simulink model "hibrido"  (R2020a)
settings: Solver=VariableStepAuto  StartTime=0.0  StopTime=3  RelTol=1e-3
values from neighbouring files (symbols this model uses):
  fd = [10/sqrt(2); 10/sqrt(2)]    [hibrido_control.m]
  Ke = 1000    [hibrido_control.m]
  Kp = wn_c^2*eye(2)    [hibrido_control.m]
  Kpf = wn_f^2    (= 16000000)    [hibrido_control.m]
  Kv = 2*xi*wn_c*eye(2)    [hibrido_control.m]
  Kvf = 2*xi*wn_f    (= 8000)    [hibrido_control.m]
  tstep = 0.2    [hibrido_control.m]
  x0 = [0.5, 1.5]    [hibrido_control.m]
  xf = [1.5, 0.5]    [hibrido_control.m]
undefined symbols (not defined in the file or in its folder): coriolis, Robot
libraries: roblocks x14
settings Model: Creator=User  LastModifiedBy=USUARIO
settings SFSimCC: CustomCodeUndefinedFunction=UseInterfaceOnly

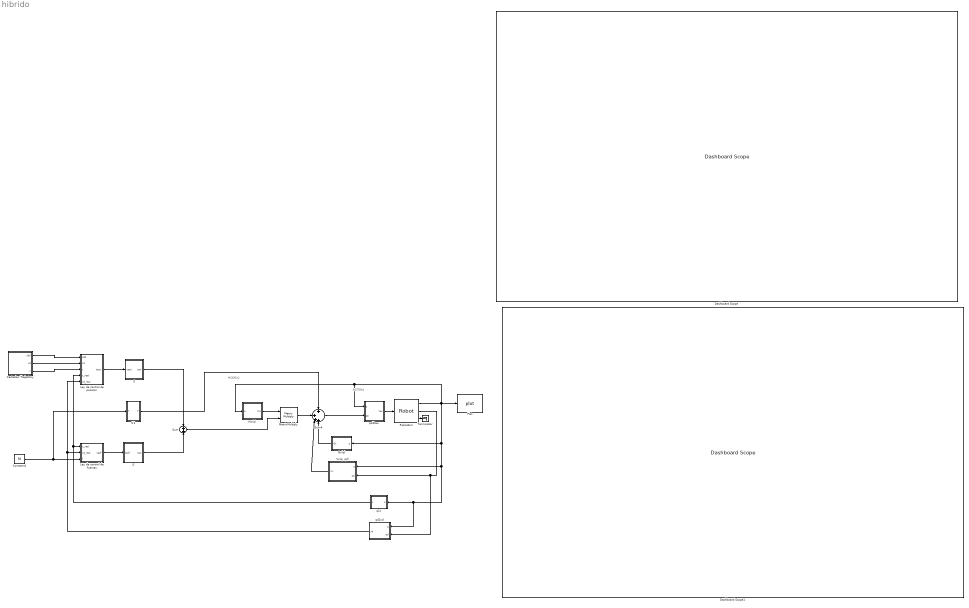
== system hibrido ==
  note: SISTEMA
  note: MODELO
  Cartesian Trajectory : Subsystem  mask{initial_x=x0, final_x=xf, t_max=tf, ts=tstep}
      mask prompts: initial_x "Initial X"; final_x "Final X"; t_max "Maximum time"; ts "Timestep"
  Constant1 : Constant  Value=fd
  Dashboard Scope : DashboardScope
  Dashboard Scope1 : DashboardScope  Ymax=13
  "Gx(q) " : Subsystem  mask{robot=Robot}
  Ley de control de fuerzas : Subsystem
  Ley de control de posicion : Subsystem
  MatrixMultiply : Product  Multiplication=Matrix(*)
  Mx(q) : Subsystem  mask{robot=Robot}
  Plot : roblocks/Arm/plot  robot=Robot  fps=30  holdplot=on
  RobotArm : roblocks/Arm/Robot  robot=Robot  q0=q0
  S : Subsystem  mask{robot=0}
  S' : Subsystem  mask{robot=0}
  S'1 : Subsystem  mask{robot=0}
  Sum : Sum  Inputs=+|+
  Sum4 : Sum  Inputs=+|+++
  Terminator : Terminator
  "Vx(q, qd)" : Subsystem  mask{robot=Robot}
  psi2tau : Subsystem  mask{robot=Robot}
  q2x : Subsystem  mask{robot=Robot}
  qd2xd : Subsystem  mask{robot=Robot}
  wires:
  RobotArm/3 -> Terminator/1
  Sum4/1 -> psi2tau/2(psi)
  RobotArm/1 -> qd2xd/1(q), q2x/1(q), "Vx(q, qd)"/1(q), "Gx(q) "/1(q), Plot/1, Mx(q)/1(q), psi2tau/1(q)
  RobotArm/2 -> qd2xd/2(qd), "Vx(q, qd)"/2(qd)
  Mx(q)/1(Mx) -> MatrixMultiply/1
  psi2tau/1(tau) -> RobotArm/1
  Cartesian Trajectory/1(xdd) -> Ley de control de posicion/1(xdd)
  Cartesian Trajectory/2(xd) -> Ley de control de posicion/2(xd)
  Cartesian Trajectory/3(x) -> Ley de control de posicion/3(x)
  q2x/1(x) -> Ley de control de posicion/4(x_real), Ley de control de fuerzas/1(x_real)
  qd2xd/1(xd) -> Ley de control de posicion/5(xd_real), Ley de control de fuerzas/2(xd_real)
  Constant1/1 -> S'1/1(f), Ley de control de fuerzas/3(f)
  Ley de control de posicion/1(taoc') -> S/1(taoc')
  Ley de control de fuerzas/1(taof') -> S'/1(taof')
  S/1(tao') -> Sum/1
  S'/1(tao') -> Sum/2
  Sum/1 -> MatrixMultiply/2
  MatrixMultiply/1 -> Sum4/2
  "Gx(q) "/1(Gx) -> Sum4/4
  "Vx(q, qd)"/1(Vx) -> Sum4/3
  S'1/1(f') -> Sum4/1

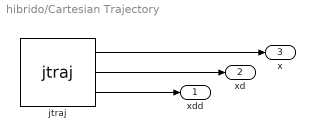
== system hibrido/Cartesian Trajectory ==
  jtraj : roblocks/Toolbox/jtraj  q0=initial_x  qf=final_x  tmax=t_max  ts=ts
  xdd : Outport  VectorParamsAs1DForOutWhenUnconnected=off
  xd : Outport  Port=2  VectorParamsAs1DForOutWhenUnconnected=off
  x : Outport  Port=3  VectorParamsAs1DForOutWhenUnconnected=off
  wires:
  jtraj/2 -> xd/1
  jtraj/1 -> x/1
  jtraj/3 -> xdd/1

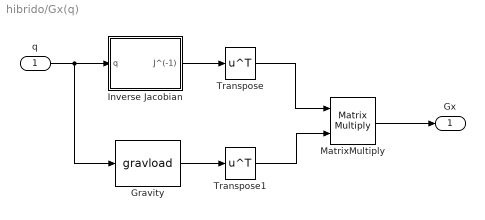
== system hibrido/Gx(q)  ==
  q : Inport
  Gravity : roblocks/Arm/gravload  robot=Robot
  Inverse Jacobian : Subsystem  mask{robot=robot}
  MatrixMultiply : Product  Multiplication=Matrix(*)
  Transpose : Math  Operator=transpose  SignedPower=on  SaturateOnIntegerOverflow=on
  Transpose1 : Math  Operator=transpose  SignedPower=on  SaturateOnIntegerOverflow=on
  Gx : Outport  VectorParamsAs1DForOutWhenUnconnected=off
  wires:
  q/1 -> Gravity/1, Inverse Jacobian/1(q)
  Inverse Jacobian/1(J^(-1)) -> Transpose/1
  Transpose/1 -> MatrixMultiply/1
  Gravity/1 -> Transpose1/1
  MatrixMultiply/1 -> Gx/1
  Transpose1/1 -> MatrixMultiply/2

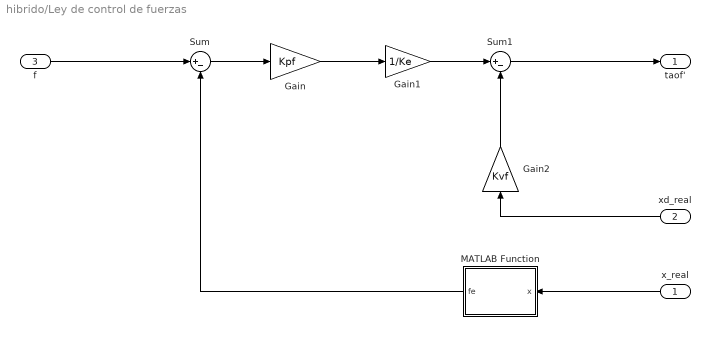
== system hibrido/Ley de control de fuerzas ==
  x_real : Inport
  xd_real : Inport  Port=2
  f : Inport  Port=3
  Gain : Gain  Gain=Kpf
  Gain1 : Gain  Gain=1/Ke
  Gain2 : Gain  Gain=Kvf
  MATLAB Function : MATLAB Function  TreatAsAtomicUnit=on
  Sum : Sum  Inputs=|+-
  Sum1 : Sum  Inputs=|+-
  taof' : Outport
  wires:
  Gain1/1 -> Sum1/1
  Gain2/1 -> Sum1/2
  Sum/1 -> Gain/1
  Sum1/1 -> taof'/1
  Gain/1 -> Gain1/1
  x_real/1 -> MATLAB Function/1(x)
  xd_real/1 -> Gain2/1
  f/1 -> Sum/1
  MATLAB Function/1(fe) -> Sum/2

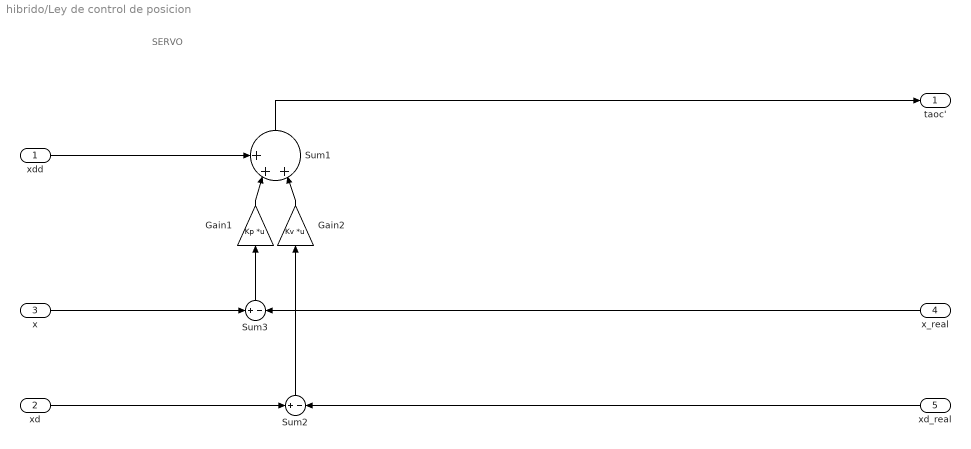
== system hibrido/Ley de control de posicion ==
  note: SERVO
  xdd : Inport
  xd : Inport  Port=2
  x : Inport  Port=3
  x_real : Inport  Port=4
  xd_real : Inport  Port=5
  Gain1 : Gain  Gain=Kp  Multiplication=Matrix(K*u)
  Gain2 : Gain  Gain=Kv  Multiplication=Matrix(K*u)
  Sum1 : Sum  Inputs=+++|
  Sum2 : Sum  Inputs=+|-
  Sum3 : Sum  Inputs=+|-
  taoc' : Outport
  wires:
  xd_real/1 -> Sum2/2
  xd/1 -> Sum2/1
  Gain1/1 -> Sum1/2
  Sum3/1 -> Gain1/1
  Gain2/1 -> Sum1/3
  xdd/1 -> Sum1/1
  Sum2/1 -> Gain2/1
  Sum1/1 -> taoc'/1
  x/1 -> Sum3/1
  x_real/1 -> Sum3/2

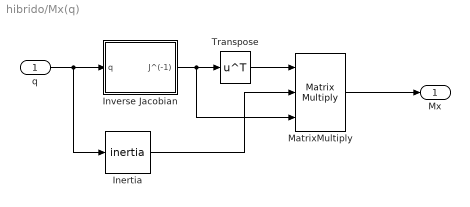
== system hibrido/Mx(q) ==
  q : Inport
  Inertia : roblocks/Arm/inertia  robot=robot
  Inverse Jacobian : Subsystem  mask{robot=robot}
  MatrixMultiply : Product  Inputs=3  Multiplication=Matrix(*)
  Transpose : Math  Operator=transpose  SignedPower=on  SaturateOnIntegerOverflow=on
  Mx : Outport  VectorParamsAs1DForOutWhenUnconnected=off
  wires:
  MatrixMultiply/1 -> Mx/1
  q/1 -> Inertia/1, Inverse Jacobian/1(q)
  Inverse Jacobian/1(J^(-1)) -> MatrixMultiply/3, Transpose/1
  Transpose/1 -> MatrixMultiply/1
  Inertia/1 -> MatrixMultiply/2

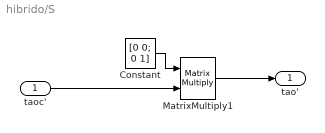
== system hibrido/S ==
  taoc' : Inport
  Constant : Constant  Value=[0 0; 0 1]
  MatrixMultiply1 : Product  Multiplication=Matrix(*)
  tao' : Outport
  wires:
  MatrixMultiply1/1 -> tao'/1
  Constant/1 -> MatrixMultiply1/1
  taoc'/1 -> MatrixMultiply1/2

== system hibrido/S' ==
  taof' : Inport
  Constant : Constant  Value=[1 0; 0 0]
  MatrixMultiply1 : Product  Multiplication=Matrix(*)
  tao' : Outport
  wires:
  MatrixMultiply1/1 -> tao'/1
  Constant/1 -> MatrixMultiply1/1
  taof'/1 -> MatrixMultiply1/2

== system hibrido/S'1 ==
  f : Inport
  Constant : Constant  Value=[1 0; 0 0]
  MatrixMultiply1 : Product  Multiplication=Matrix(*)
  f' : Outport
  wires:
  MatrixMultiply1/1 -> f'/1
  Constant/1 -> MatrixMultiply1/1
  f/1 -> MatrixMultiply1/2

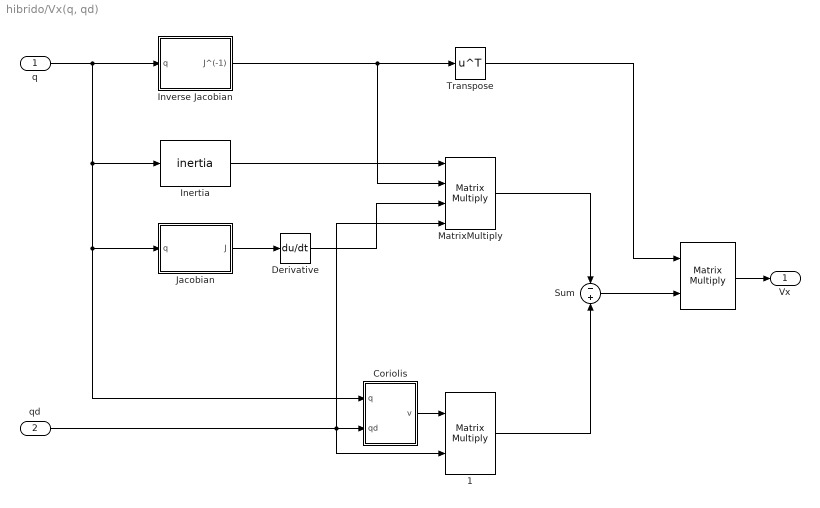
== system hibrido/Vx(q, qd) ==
  q : Inport
  qd : Inport  Port=2
  " " : Product  Multiplication=Matrix(*)
  " 1" : Product  Multiplication=Matrix(*)
  Coriolis : Subsystem  mask{robot=robot}
  Derivative : Derivative
  Inertia : roblocks/Arm/inertia  robot=robot
  Inverse Jacobian : Subsystem  mask{robot=robot}
  Jacobian : Subsystem  mask{robot=robot}
  MatrixMultiply : Product  Inputs=4  Multiplication=Matrix(*)
  Sum : Sum  Inputs=-+
  Transpose : Math  Operator=transpose  SignedPower=on  SaturateOnIntegerOverflow=on
  Vx : Outport  VectorParamsAs1DForOutWhenUnconnected=off
  wires:
  " "/1 -> Vx/1
  qd/1 -> Coriolis/2(qd), MatrixMultiply/4, " 1"/2
  q/1 -> Inverse Jacobian/1(q), Coriolis/1(q), Jacobian/1(q), Inertia/1
  Inverse Jacobian/1(J^(-1)) -> MatrixMultiply/2, Transpose/1
  Transpose/1 -> " "/1
  Jacobian/1(J) -> Derivative/1
  Inertia/1 -> MatrixMultiply/1
  Derivative/1 -> MatrixMultiply/3
  Coriolis/1(v) -> " 1"/1
  MatrixMultiply/1 -> Sum/1
  Sum/1 -> " "/2
  " 1"/1 -> Sum/2

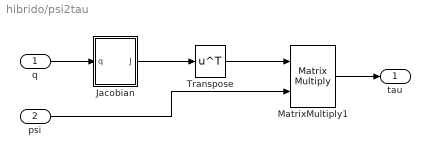
== system hibrido/psi2tau ==
  q : Inport
  psi : Inport  Port=2
  Jacobian : Subsystem  mask{robot=robot}
  MatrixMultiply1 : Product  Multiplication=Matrix(*)
  Transpose : Math  Operator=transpose  SignedPower=on  SaturateOnIntegerOverflow=on
  tau : Outport  VectorParamsAs1DForOutWhenUnconnected=off
  wires:
  q/1 -> Jacobian/1(q)
  Jacobian/1(J) -> Transpose/1
  Transpose/1 -> MatrixMultiply1/1
  MatrixMultiply1/1 -> tau/1
  psi/1 -> MatrixMultiply1/2

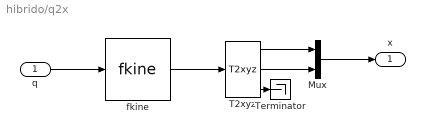
== system hibrido/q2x ==
  q : Inport
  Mux : Mux  Inputs=2
  T2xyz : roblocks/Toolbox/T2xyz
  Terminator : Terminator
  fkine : roblocks/Arm/fkine  robot=robot
  x : Outport  VectorParamsAs1DForOutWhenUnconnected=off
  wires:
  q/1 -> fkine/1
  fkine/1 -> T2xyz/1
  Mux/1 -> x/1
  T2xyz/1 -> Mux/1
  T2xyz/2 -> Mux/2
  T2xyz/3 -> Terminator/1

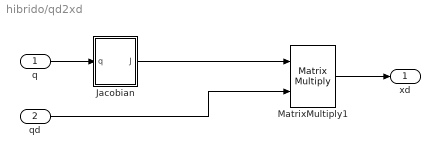
== system hibrido/qd2xd ==
  q : Inport
  qd : Inport  Port=2
  Jacobian : Subsystem  mask{robot=robot}
  MatrixMultiply1 : Product  Multiplication=Matrix(*)
  xd : Outport  VectorParamsAs1DForOutWhenUnconnected=off
  wires:
  q/1 -> Jacobian/1(q)
  Jacobian/1(J) -> MatrixMultiply1/1
  MatrixMultiply1/1 -> xd/1
  qd/1 -> MatrixMultiply1/2

== system hibrido/Gx(q) /Inverse Jacobian ==
  q : Inport
  Invert Jacobian : MATLABFcn  MATLABFcn=[u(1:robot.n)',u(6+1:6+robot.n)']^(-1)  OutputDimensions=[robot.n, robot.n]  Output1D=off
  jacobn : roblocks/Arm/jacobn  robot=robot
  J^(-1) : Outport  VectorParamsAs1DForOutWhenUnconnected=off
  wires:
  jacobn/1 -> Invert Jacobian/1
  q/1 -> jacobn/1
  Invert Jacobian/1 -> J^(-1)/1

== system hibrido/Mx(q)/Inverse Jacobian ==
  q : Inport
  Invert Jacobian : MATLABFcn  MATLABFcn=[u(1:robot.n)',u(6+1:6+robot.n)']^(-1)  OutputDimensions=[robot.n, robot.n]  Output1D=off
  jacobn : roblocks/Arm/jacobn  robot=robot
  J^(-1) : Outport  VectorParamsAs1DForOutWhenUnconnected=off
  wires:
  Invert Jacobian/1 -> J^(-1)/1
  q/1 -> jacobn/1
  jacobn/1 -> Invert Jacobian/1

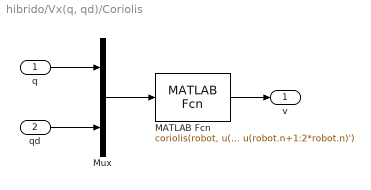
== system hibrido/Vx(q, qd)/Coriolis ==
  q : Inport
  qd : Inport  Port=2
  MATLAB Fcn : MATLABFcn  MATLABFcn=coriolis(robot, u(1:robot.n)', u(robot.n+1:2*robot.n)')  OutputDimensions=[robot.n, robot.n]  Output1D=off
  Mux : Mux  Inputs=2
  v : Outport  VectorParamsAs1DForOutWhenUnconnected=off
  wires:
  qd/1 -> Mux/2
  MATLAB Fcn/1 -> v/1
  Mux/1 -> MATLAB Fcn/1
  q/1 -> Mux/1

== system hibrido/Vx(q, qd)/Inverse Jacobian ==
  q : Inport
  Invert Jacobian : MATLABFcn  MATLABFcn=[u(1:robot.n)',u(6+1:6+robot.n)']^(-1)  OutputDimensions=[robot.n, robot.n]  Output1D=off
  jacobn : roblocks/Arm/jacobn  robot=robot
  J^(-1) : Outport  VectorParamsAs1DForOutWhenUnconnected=off
  wires:
  jacobn/1 -> Invert Jacobian/1
  q/1 -> jacobn/1
  Invert Jacobian/1 -> J^(-1)/1

== system hibrido/Vx(q, qd)/Jacobian ==
  q : Inport
  Slice : MATLABFcn  MATLABFcn=[u(1:robot.n)',u(6+1:6+robot.n)']  OutputDimensions=[robot.n, robot.n]  Output1D=off
  jacobn : roblocks/Arm/jacobn  robot=robot
  J : Outport  VectorParamsAs1DForOutWhenUnconnected=off
  wires:
  q/1 -> jacobn/1
  jacobn/1 -> Slice/1
  Slice/1 -> J/1

== system hibrido/psi2tau/Jacobian ==
  q : Inport
  Slice : MATLABFcn  MATLABFcn=[u(1:robot.n)',u(6+1:6+robot.n)']  OutputDimensions=[robot.n, robot.n]  Output1D=off
  jacobn : roblocks/Arm/jacobn  robot=robot
  J : Outport  VectorParamsAs1DForOutWhenUnconnected=off
  wires:
  q/1 -> jacobn/1
  jacobn/1 -> Slice/1
  Slice/1 -> J/1

== system hibrido/qd2xd/Jacobian ==
  q : Inport
  Slice : MATLABFcn  MATLABFcn=[u(1:robot.n)',u(6+1:6+robot.n)']  OutputDimensions=[robot.n, robot.n]  Output1D=off
  jacobn : roblocks/Arm/jacobn  robot=robot
  J : Outport  VectorParamsAs1DForOutWhenUnconnected=off
  wires:
  q/1 -> jacobn/1
  jacobn/1 -> Slice/1
  Slice/1 -> J/1

== matlab function hibrido/Ley de control de fuerzas/MATLAB Function ==
  data: x input; fe output
function fe = ModeloFuerza(x)
%   PARED   %
a = -1;     
b = 2;  
c = 1;

%   DEFINO LIMITES  %
y_limite =(x(1)*a+b)/c;
x_limite = (c*x(2)-b)/a;
ke = 1000;          % cte. de rigidez


if((x(1)<x_limite)&&(x(2)<y_limite))  % Analizo si no pase la pared
    fe=[0 0]';
    
% Si paso la pared...
else
    %   distancia = |ax + b - cy|/sqrt(a^2+c^2)
    distancia = abs(a*x(1)+b-c*x(2))/sqrt(a^2+c^2);             % Calculo distancia del punto a la recta (pared)
    fe = [distancia*(ke/sqrt(2)) distancia*(ke/sqrt(2))]';  %  
end
